simulink model "nonPred_TestModel_FCEV_ECMS_and_Battery_age"  (R2022b)
settings: Solver=ode4  StartTime=1  StopTime=DrvCycLen  FixedStep=Auto  RelTol=1e-3  EnableMultiTasking=on
values from neighbouring files (symbols this model uses):
  Bat_eff_chg_average = 0.969    [FCEV_original_data.mat]
  Bat_eff_dis_average = 0.9632    [FCEV_original_data.mat]
  Bat_end_of_life_percent = 20    [FCEV_original_data.mat]
  Bat_I_chg_max = -120    [FCEV_original_data.mat]
  Bat_I_dis_max = 200    [FCEV_original_data.mat]
  Bat_nom_Ic = 2.5    [FCEV_original_data.mat]
  Bat_nom_SOC = 0.35    [FCEV_original_data.mat]
  Bat_nom_temp_oC = 25    [FCEV_original_data.mat]
  Bat_num_pa = 9    [FCEV_original_data.mat]
  Bat_num_se = 97    [FCEV_original_data.mat]
  Bat_ori_C1_chg_F = [397.526659684 455.660832136 435.08783522 460.845064365 457.605812374 417.289828504 416.373906992 359.741413056 321.561704819 1109.14132554 1165.67733205 1135.97600211 ... (72 elements, 9x8)]    [FCEV_original_data.mat]
  Bat_ori_C1_dis_F = [187.121968588 287.083505726 346.448009002 395.529439835 387.517274826 389.973134196 432.856765051 486.92921923 512.158935268 425.990733989 614.68708868 771.472592368 ... (72 elements, 9x8)]    [FCEV_original_data.mat]
  Bat_ori_C2_chg_F = [8748.48589695 7773.35875681 9404.86567646 8934.73981058 8290.58671366 7592.78422269 7759.44623103 7396.59043829 6151.35152293 16187.7227039 11721.8480541 13157.8579836 ... (72 elements, 9x8)]    [FCEV_original_data.mat]
  Bat_ori_C2_dis_F = [2939.81325553 4590.73311898 5504.93546413 5887.5077374 6534.37836712 7765.46899768 10584.7751706 10372.0508438 9238.72693885 5207.86390693 7911.43744944 8879.62137571 ... (72 elements, 9x8)]    [FCEV_original_data.mat]
  Bat_ori_cap_max_Ah = 20.7    [Config_c221218.m]    (also in Config_c230117.m; Config_c230321.m; FCEV_original_data.mat)
  Bat_ori_dUdt4 = [-0.303773584906 -0.249056603774 -0.115094339623 -0.0396226415094 0.0396226415094 0.0641509433962 0.107547169811 0.111320754717 0.0415094339623 0.0547169811321 0.130188679245]    [FCEV_original_data.mat]
  Bat_ori_R0_chg_O = [0.0771669453735 0.0731809311402 0.0726556782939 0.0729965156794 0.0731758310684 0.0742031005051 0.0721266921026 0.0714211058078 0.0714186176143 0.0374124505155 0.0354566732504 0.0345430657188 ... (72 elements, 9x8)]    [FCEV_original_data.mat]
  Bat_ori_R0_dis_O = [0.0819458671157 0.0812429476608 0.0803749674507 0.0805513601722 0.0838629023857 0.0850797840015 0.0829875518672 0.0826388888889 0.0812514106148 0.0428124986417 0.0424658903711 0.0428572670451 ... (72 elements, 9x8)]    [FCEV_original_data.mat]
  Bat_ori_R1_chg_O = [0.114339870884 0.105392753268 0.104421193553 0.109821896183 0.114868279838 0.123333154908 0.129174812826 0.149917249373 0.174896487845 0.0420560161846 0.0390948352938 0.0370122837364 ... (72 elements, 9x8)]    [FCEV_original_data.mat]
  Bat_ori_R1_dis_O = [0.304806399643 0.213604089624 0.171463520004 0.151183840498 0.140630862434 0.128795299077 0.116857791733 0.112567113582 0.106368362501 0.0943235089866 0.0730697254134 0.0611414736086 ... (72 elements, 9x8)]    [FCEV_original_data.mat]
  Bat_ori_R2_chg_O = [0.134518959939 0.17565045702 0.161100627268 0.189032232545 0.205639040497 0.226170473035 0.223651875822 0.181765694192 0.212966950836 0.073628872144 0.0788540822416 0.0792414571734 ... (72 elements, 9x8)]    [FCEV_original_data.mat]
  Bat_ori_R2_dis_O = [0.354968099904 0.285293035102 0.286338708953 0.298763853987 0.248762838155 0.178586175471 0.129047399775 0.188406991173 0.174494800676 0.131839238891 0.123225430215 0.132069033134 ... (72 elements, 9x8)]    [FCEV_original_data.mat]
  Bat_ori_SOC2 = [0 0.001 0.002 0.003 0.004 0.005 0.006 0.007 0.008 0.009 0.01 0.011 ... (1001 elements, 1x1001)]    [FCEV_original_data.mat]
  Bat_ori_SOC4 = [-0.00598301069999 0.0920117618231 0.190864167279 0.289083557951 0.387343788287 0.485011843502 0.5850485992 0.678163031937 0.774810095565 0.876684636119 0.972739524626]    [FCEV_original_data.mat]
  Bat_ori_Uoc_chg_V = [2.4478 2.54923264342 2.6007 2.6383 2.66953057366 2.69636321708 2.7197 2.74042850391 2.75906114733 2.77619379074 2.792 2.80675907757 ... (1001 elements, 1x1001)]    [FCEV_original_data.mat]
  Bat_ori_Uoc_dis_V = [1.9998 2.03916768329 2.24724374236 2.39700902919 2.48767431602 2.5476 2.5882 2.6202 2.64771773167 2.6719 2.6933 2.71251566192 ... (1001 elements, 1x1001)]    [FCEV_original_data.mat]
  Bat_ori_Uoc_V = [2.2238 2.29420016335 2.42397187118 2.5176545146 2.57860244484 2.62198160854 2.65395 2.68031425195 2.7033894395 2.72404689537 2.74265 2.75963736975 ... (1001 elements, 1x1001)]    [FCEV_original_data.mat]
  Bat_single_capacity_nom_Ah = 2.3    [FCEV_original_data.mat]
  Bat_SOC_cs_max = 0.4    [FCEV_original_data.mat]
  Bat_SOC_cs_min = 0.2    [FCEV_original_data.mat]
  Bat_SOC_ini = 0.3    [Config_c22100601.m]    (also in Config_c22100701.m; FCEV_original_data.mat = 0.45)
  Bat_SOC_max = 0.9    [FCEV_original_data.mat]
  Bat_SOC_min = 0.3    [FCEV_original_data.mat]
  Bat_temp_amb_oC = 25    [FCEV_original_data.mat]
  Bat_temp_cool_oC = 25    [FCEV_original_data.mat]
  BattSocInit = 0.9    [Config_c221112.m]    (also in Config_c221127.m = 0.3; Config_c221218.m = 0.3; Config_c230117.m = 0.8; Config_c230321.m = 0.8)
  BattSocLowerLimit = 0.25    [Config_c221112.m]    (also in Config_c221127.m = 0.3; Config_c221218.m = 0.3; Config_c230117.m = 0.3; Config_c230321.m = 0.3)
  DCAC_eff = 0.95    [FCEV_original_data.mat]
  DCDC_ori_eff = [0.95 0.96 0.97 0.976 0.98 0.978 0.973 0.962]    [FCEV_original_data.mat]
  DCDC_ori_eff_avg = 0.9686    [FCEV_original_data.mat]
  DCDC_ori_power_kW = [0 10 20 30 40 50 60 70]    [FCEV_original_data.mat]
  FC_fuel_mass_ini_kg = 10    [FCEV_original_data.mat]
  FC_ori_eff = [0.1 0.33 0.492 0.533 0.559 0.596 0.591 0.562 0.508]    [FCEV_original_data.mat]
  FC_ori_fuel_rate_gps = [0 0.0505050505051 0.0846883468835 0.117260787992 0.149075730471 0.279642058166 0.423011844332 0.593119810202 0.820209973753]    [FCEV_original_data.mat]
  FC_ori_power_kW = [0 2 5 7.5 10 20 30 40 50]    [FCEV_original_data.mat]
  FC_power_max_kW = 50    [FCEV_original_data.mat]
  FC_power_min_kW = 0    [FCEV_original_data.mat]
  HydpriceRmb = 30    [Config_c221127.m]    (also in Config_c221218.m; Config_c230117.m; Config_c230321.m)
  m = Time_sample    [Config_c22100601.m]    (also in Config_c22100701.m)
  MC_eff_brk_average = 0.810578512397    [FCEV_original_data.mat]
  MC_eff_dri_average = 0.810578512397    [FCEV_original_data.mat]
  MC_inertia = 0.06    [FCEV_original_data.mat]
  MC_ori_eff = [0.7 0.78 0.85 0.86 0.81 0.82 0.79 0.78 0.78 0.78 0.78 0.7 ... (231 elements, 11x21)]    [FCEV_original_data.mat]
  MC_ori_power_brk_req_kW = [0 -28.3912930389 -56.7825860779 -85.1738791168 -113.565172156 -141.956465195 -170.347758234 -198.739051273 -227.130344311 -255.52163735 -283.912930389 0 ... (121 elements, 11x11)]    [FCEV_original_data.mat]
  MC_ori_power_dri_req_kW = [0 0 0 0 0 0 0 0 0 0 0 0 ... (121 elements, 11x11)]    [FCEV_original_data.mat]
  MC_ori_spd_rpm = [0 1000 2000 3000 4000 5000 6000 7000 8000 9000 10000]    [FCEV_original_data.mat]
  MC_ori_trq_brk_max_Nm = [-271.1368 -271.1368 -271.1368 -237.5159 -178.1369 -142.4824 -118.7579 -101.8119 -89.0685 -79.172 -71.1734]    [FCEV_original_data.mat]
  MC_ori_trq_brk_Nm = [-271.136848522 -244.02316367 -216.909478817 -189.795793965 -162.682109113 -135.568424261 -108.454739409 -81.3410545565 -54.2273697044 -27.1136848522 0]    [FCEV_original_data.mat]
  MC_ori_trq_dri_max_Nm = [271.1368 271.1368 271.1368 237.5159 178.1369 142.4824 118.7579 101.8119 89.0685 79.172 71.1734]    [FCEV_original_data.mat]
  MC_ori_trq_dri_Nm = [0 27.1136848522 54.2273697044 81.3410545565 108.454739409 135.568424261 162.682109113 189.795793965 216.909478817 244.02316367 271.136848522]    [FCEV_original_data.mat]
  MC_ori_trq_Nm = [-271.136848522 -244.02316367 -216.909478817 -189.795793965 -162.682109113 -135.568424261 -108.454739409 -81.3410545565 -54.2273697044 -27.1136848522 0 27.1136848522 ... (21 elements, 1x21)]    [FCEV_original_data.mat]
  MC_power_max_kW = 75    [FCEV_original_data.mat]
  MC_spd_max_rpm = 10000    [FCEV_original_data.mat]
  MC_spd_min_rpm = 0    [FCEV_original_data.mat]
  MC_spd_scale = 1    [FCEV_original_data.mat]
  MC_trq_scale = 1    [FCEV_original_data.mat]
  MC_U_min_V = 120    [FCEV_original_data.mat]
  Road_u = 0.75    [FCEV_original_data.mat]
  tDegTable = [zeros(1,3),linspace(0,0.13,47)]    [Config_c221127.m]    (also in Config_c221218.m; Config_c230117.m; Config_c230321.m)
  usd2rmb = 7.116    [Config_c22100601.m]    (also in Config_c22100701.m; Config_c221106.m = 6; Config_c221112.m = 6; Config_c221127.m = 6)
  Veh_air_density_kgpm2 = 1.2    [FCEV_original_data.mat]
  Veh_brk_front = [1 0.6 0.608 0.61 0.618 0.624 0.636 0.645 0.655]    [FCEV_original_data.mat]
  Veh_brk_z = [0.1 0.2 0.3 0.4 0.5 0.6 0.7 0.8 0.9]    [FCEV_original_data.mat]
  Veh_brk_z_max = 0.7    [FCEV_original_data.mat]
  Veh_brk_z_min = 0.1    [FCEV_original_data.mat]
  Veh_coeff_drag = 0.312    [FCEV_original_data.mat]
  Veh_coeff_roll = 0.00863    [FCEV_original_data.mat]
  Veh_final_drive_inertia = 0.1105    [FCEV_original_data.mat]
  Veh_final_drive_ratio = 3.47    [FCEV_original_data.mat]
  Veh_frontal_area_m2 = 2.06    [FCEV_original_data.mat]
  Veh_gravity_acc_ms2 = 9.81    [FCEV_original_data.mat]
  Veh_mass_cargo_kg = 113    [FCEV_original_data.mat]
  Veh_mass_curb_kg = 1157    [FCEV_original_data.mat]
  Veh_mech_eff = 0.9    [FCEV_original_data.mat]
  Veh_rotary_mass_conversion_factor = 1.05    [FCEV_original_data.mat]
  Veh_size_cg_height_m = 0.53    [FCEV_original_data.mat]
  Veh_wheel_inertia = 3.1039    [FCEV_original_data.mat]
  Veh_wheel_radius_m = 0.313    [FCEV_original_data.mat]
  Veh_wt_frac_front = 0.5    [FCEV_original_data.mat]
undefined symbols (not defined in the file or in its folder): Bat_ori_temp
libraries: autolibshared x1
(part 1 of 3)
settings Model: Creator=阿瑞的PC  LastModifiedBy=xuupp
settings SolverCC: AlgebraicLoopSolver=TrustRegion
settings DataIOCC: LimitDataPoints=on  SaveFormat=Array  ReturnWorkspaceOutputs=off
settings OptimizationCC: LifeSpan=inf
settings DebuggingCC: MaxConsecutiveZCsMsg=none  SolverPrmCheckMsg=warning  UnconnectedInputMsg=warning  UnconnectedOutputMsg=warning  UnconnectedLineMsg=warning  SFUnexpectedBacktrackingDiag=warning  SFNoUnconditionalDefaultTransitionDiag=warning  SFExecutionAtInitializationDiag=none  SFMachineParentedDataDiag=warning  ArithmeticOperatorsInVariantConditions=warning
settings HardwareCC: ProdBitPerPointer=32  ProdBitPerSizeT=32  ProdBitPerPtrDiffT=32  ProdLargestAtomicFloat=None  ProdIntDivRoundTo=Undefined  ProdEndianess=Unspecified  ProdWordSize=32  ProdHWDeviceType=32-bit Generic
settings ModelReferenceCC: EnableRefExpFcnMdlSchedulingChecks=on  PropagateSignalLabelsOutOfModel=off
settings SFSimCC: SimUseLocalCustomCode=off  CustomCodeUndefinedFunction=UseInterfaceOnly
settings RTWCC: RTWUseLocalCustomCode=off  DLArmComputeVersion=19.05
settings CodeAppCC: StateflowObjectComments=on
settings GRTTargetCC: TargetLangStandard=C89/C90 (ANSI)
settings ConfigComp: CovMetricSettings=dw  CovSaveCumulativeToWorkspaceVar=on  CovSaveSingleToWorkspaceVar=on  CovExternalEMLEnable=off  CovSFcnEnable=off
settings SimscapeCC: SimscapeNormalizeSystem=off
settings ConfigurationSet: Description=SimMechanics 2G

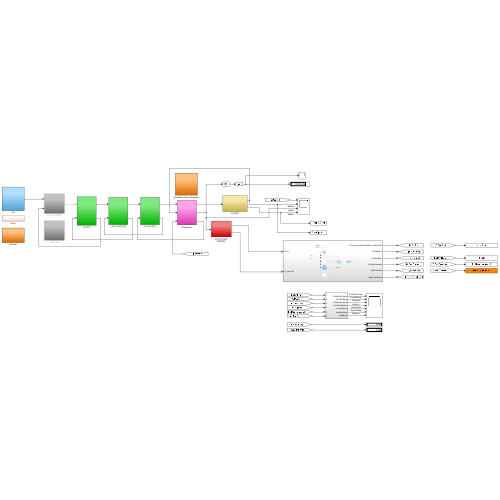
[thumbnail: Simulink's stored preview of the top-level diagram]
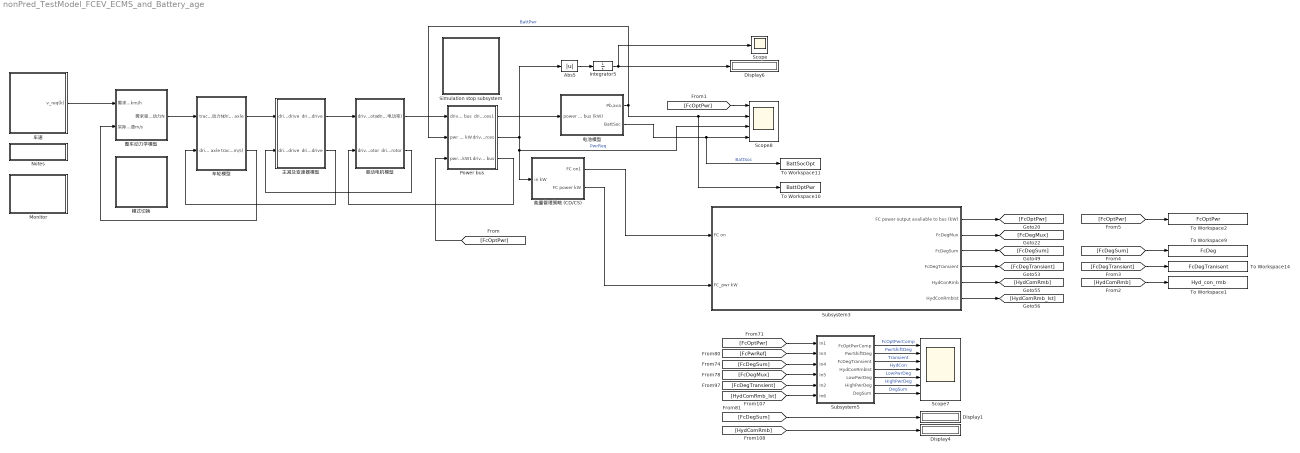
== system nonPred_TestModel_FCEV_ECMS_and_Battery_age ==
  Abs5 : Abs  SaturateOnIntegerOverflow=off
  Display1 : Display
  Display4 : Display
  Display6 : Display
  Integrator5 : Integrator
  Monitor : Subsystem
  Notes : Subsystem
  Power bus : Subsystem
  Scope : Scope
  Scope7 : Scope  NumInputPorts=7
  Scope8 : Scope  NumInputPorts=4
  Simulation stop subsystem : Subsystem
  Subsystem3 : Subsystem
  Subsystem5 : Subsystem
  To Workspace1 : ToWorkspace  VariableName=Hyd_con_rmb  SampleTime=-1
  To Workspace10 : ToWorkspace  VariableName=BattOptPwr  SampleTime=-1
  To Workspace11 : ToWorkspace  VariableName=BattSocOpt  SampleTime=-1
  To Workspace14 : ToWorkspace  VariableName=FcDegTranisent  SampleTime=-1
  To Workspace2 : ToWorkspace  VariableName=FcOptPwr  SampleTime=-1
  To Workspace9 : ToWorkspace  VariableName=FcDeg  SampleTime=-1
  主减及变速器模型 : Subsystem
  整车动力学模型 : Subsystem
  模式切换 : Subsystem
  电池模型 : Subsystem
  能量管理策略 (CD/CS) : Subsystem
  车轮模型 : Subsystem
  车速 : Subsystem
  驱动电机模型 : Subsystem
  wires:
  主减及变速器模型/1(drive torque (Nm) speed (rad/s) brike torque (Nm) req'd at input side of final drive) -> 驱动电机模型/1(drive torque (Nm) speed (rad/s) brake torque (Nm) req'd at motor)
  驱动电机模型/2(drive torque (Nm) brake torque (Nm) speed avail (rad/s) avail. at rotor) -> 主减及变速器模型/2(drive torque (Nm) brake torque (Nm) speed avail (rad/s) at input side of final drive)
  主减及变速器模型/2(drive torque (Nm) brake torque (Nm) speed avail (rad/s) at output side of final drive) -> 车轮模型/2("drive torque (Nm) brake torque (Nm) speed (rad/s) available from drivetrain into axle ")
  车轮模型/2(tractive force (N) brake force (N) linear speed achievable (m/s)) -> 整车动力学模型/2(实际车辆驱动力N 制动力N 和车速m/s)
  整车动力学模型/1(需求驱动力N 目标车速m/s 需求制动力N) -> 车轮模型/1("tractive force, brake force and speed req'd of tire/road interface 需求驱动力N 目标车速m/s 需求制动力N")
  电池模型/1(Pb,ava) -> To Workspace10/1, Scope8/2, Power bus/2(pwr availible from battery kW)  "BattPwr"
  车轮模型/1(drive torque (Nm) speed (rad/s) brake torque (Nm) req'd from drivetrain into axle) -> 主减及变速器模型/1(drive torque (Nm) speed (rad/s) brake torque (Nm) req'd at output side of final drive)
  车速/1(v_req(k)) -> 整车动力学模型/1(需求车速 km/h)
  能量管理策略 (CD/CS)/2(FC power kW) -> Subsystem3/2("FC_pwr kW ")
  能量管理策略 (CD/CS)/1(FC on1) -> Subsystem3/1(FC on)
  Power bus/1(drive power (kW)/brake power (kW) req from power sources1) -> 电池模型/1(power req'd into bus (kW))
  Power bus/3(drive power (kW) brake power (kW) availableat power bus) -> 驱动电机模型/2(drive power (kW) brake power (kW) input available motor)
  Power bus/2(drive power (kW)/brake power (kW) req from power sources) -> Scope8/3, 能量管理策略 (CD/CS)/1(in kW), Abs5/1  "PwrReq"
  驱动电机模型/1(drive power (kW) brake power (kW) req'd motor input power (电功率)) -> Power bus/1(drive power (kW) brake power (kW) req at power bus)
  Abs5/1 -> Integrator5/1
  Integrator5/1 -> Display6/1, Scope/1
  电池模型/2(BattSoc) -> To Workspace11/1, Scope8/4  "BattSoc"
  Subsystem3/6(HydConRmbIst) -> [HydComRmb_Ist]
  Subsystem3/5(HydConRmb) -> [HydComRmb]
  Subsystem3/4(FcDegTransient) -> [FcDegTransient]
  Subsystem3/2(FcDegMux) -> [FcDegMux]
  Subsystem3/1(FC power output avaliable to bus (kW)) -> [FcOptPwr]
  Subsystem3/3(FcDegSum) -> [FcDegSum]
  [FcOptPwr] -> Power bus/3(pwr availible from FC kW1)
  [FcOptPwr] -> Scope8/1
  [FcOptPwr] -> Subsystem5/1(In1)
  [HydComRmb_Ist] -> Subsystem5/6(In6)
  [FcDegTransient] -> Subsystem5/5(In2)
  Subsystem5/5(LowPwrDeg) -> Scope7/5  "LowPwrDeg"
  Subsystem5/7(DegSum) -> Scope7/7  "DegSum"
  Subsystem5/2(PwrShiftDeg) -> Scope7/2  "PwrShiftDeg"
  Subsystem5/4(HydConRmbIst) -> Scope7/4  "HydCon"
  Subsystem5/6(HighPwrDeg) -> Scope7/6  "HighPwrDeg"
  [FcDegMux] -> Subsystem5/4(In5)
  [FcPwrRef] -> Subsystem5/2(In3)
  Subsystem5/3(FcDegTransient) -> Scope7/3  "Transient"
  [FcDegSum] -> Subsystem5/3(In4)
  Subsystem5/1(FcOptPwrComp) -> Scope7/1  "FcOptPwrComp"
  [HydComRmb] -> Display4/1
  [FcDegSum] -> Display1/1
  [HydComRmb] -> To Workspace1/1
  [FcDegTransient] -> To Workspace14/1
  [FcDegSum] -> To Workspace9/1
  [FcOptPwr] -> To Workspace2/1

== system nonPred_TestModel_FCEV_ECMS_and_Battery_age/Monitor ==
  note: 燃料电池模块
  note: 电池模块
  note: Power bus
  note: 电机模块
  note: 车速模块
  Display{,1..7} (8 alike) : Display
  Scope : Scope
  wires:
  [Trip_distance_travelled_km] -> Display/1
  [MC_power_dri_req_kW] -> Display1/1
  [MC_power_brk_req_kW] -> Display2/1
  [PS_power_req_kW] -> Display3/1
  [Bat_charge_sustaining_on] -> Display4/1
  [Bat_SOC] -> Scope/1, Display5/1
  [FC_fuel_rate_gps] -> Display6/1
  [FC_fuel_consume_kg] -> Display7/1

== system nonPred_TestModel_FCEV_ECMS_and_Battery_age/Notes ==
  note: Notes:
      | #1:涉及单位换算的模块统一使用紫色底色；

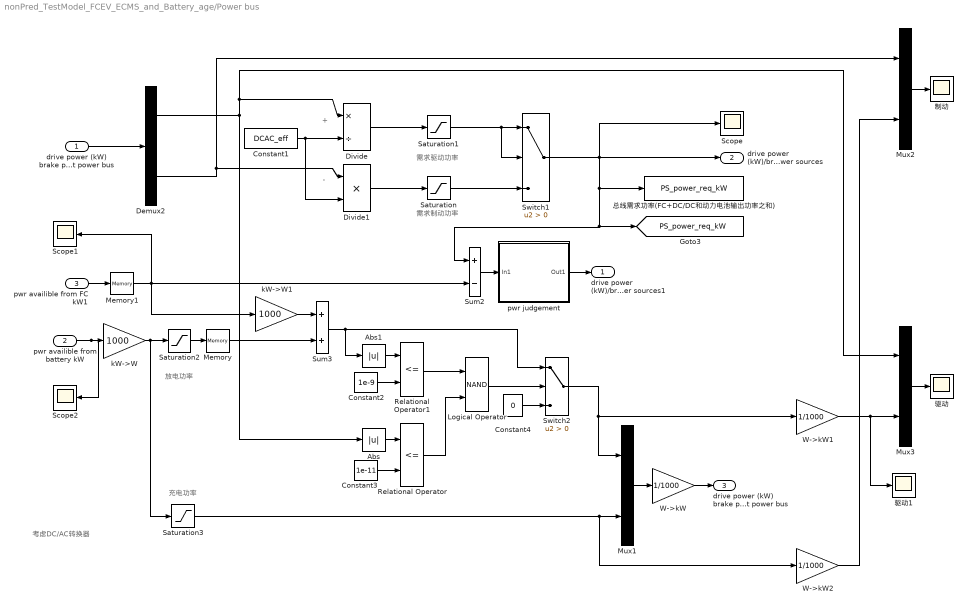
== system nonPred_TestModel_FCEV_ECMS_and_Battery_age/Power bus ==
  note: 充电功率
  note: 放电功率
  note: 考虑DC/AC转换器
  note: -
  note: +
  note: 需求制动功率
  note: 需求驱动功率
  drive power (kW) brake power (kW) req at power bus : Inport
  pwr availible from battery kW : Inport  Port=2
  pwr availible from FC kW1 : Inport  Port=3
  Abs : Abs  SaturateOnIntegerOverflow=off
  Abs1 : Abs  SaturateOnIntegerOverflow=off
  Constant1 : Constant  Value=DCAC_eff
  Constant2 : Constant  Value=1e-9
  Constant3 : Constant  Value=1e-11
  Constant4 : Constant  Value=0
  Demux2 : Demux  Outputs=2
  Divide : Product  Inputs=*/
  Divide1 : Product  Inputs=**
  Logical Operator : Logic  Operator=NAND  AllPortsSameDT=off  OutDataTypeStr=boolean
  Memory : Memory  InheritSampleTime=on
  Memory1 : Memory  InheritSampleTime=on
  Mux1 : Mux  Inputs=2
  Mux2 : Mux  Inputs=2
  Mux3 : Mux  Inputs=2
  Relational Operator : RelationalOperator  Operator=<=  OutDataTypeStr=boolean  InputSameDT=off
  Relational Operator1 : RelationalOperator  Operator=<=  OutDataTypeStr=boolean  InputSameDT=off
  Saturation : Saturate  UpperLimit=0  LowerLimit=-inf
  Saturation1 : Saturate  UpperLimit=inf  LowerLimit=0
  Saturation2 : Saturate  UpperLimit=inf  LowerLimit=0
  Saturation3 : Saturate  UpperLimit=0  LowerLimit=-inf
  Scope : Scope
  Scope1 : Scope
  Scope2 : Scope
  Sum2 : Sum  Inputs=+-
  Sum3 : Sum
  Switch1 : Switch  Criteria=u2 > Threshold  SaturateOnIntegerOverflow=off  InputSameDT=off
  Switch2 : Switch  Criteria=u2 > Threshold  SaturateOnIntegerOverflow=off  InputSameDT=off
  W->kW : Gain  Gain=1/1000
  W->kW1 : Gain  Gain=1/1000
  W->kW2 : Gain  Gain=1/1000
  kW->W : Gain  Gain=1000
  kW->W1 : Gain  Gain=1000
  pwr judgement : Subsystem
  制动 : Scope
  总线需求功率(FC+DC/DC和动力电池输出功率之和) : ToWorkspace  VariableName=PS_power_req_kW  SampleTime=-1
  驱动 : Scope
  驱动1 : Scope
  drive power (kW)/brake power (kW) req from power sources1 : Outport
  drive power (kW)/brake power (kW) req from power sources : Outport  Port=2
  drive power (kW) brake power (kW) availableat power bus : Outport  Port=3
  tag scope: PS_power_req_kW=global
  wires:
  Abs1/1 -> Relational Operator1/1
  Constant2/1 -> Relational Operator1/2
  Constant1/1 -> Divide1/2, Divide/2
  Divide/1 -> Saturation1/1
  Divide1/1 -> Saturation/1
  drive power (kW) brake power (kW) req at power bus/1 -> Demux2/1
  Demux2/2 -> Mux2/1, Divide1/1
  Saturation1/1 -> Switch1/2, Switch1/1
  Switch1/1 -> drive power (kW)/brake power (kW) req from power sources/1, 总线需求功率(FC+DC/DC和动力电池输出功率之和)/1, Sum2/1, [PS_power_req_kW], Scope/1
  W->kW/1 -> drive power (kW) brake power (kW) availableat power bus/1
  Saturation/1 -> Switch1/3
  Mux2/1 -> 制动/1
  Mux3/1 -> 驱动/1
  W->kW1/1 -> 驱动1/1, Mux3/2
  W->kW2/1 -> Mux2/2
  Sum2/1 -> pwr judgement/1(In1)
  pwr judgement/1(Out1) -> drive power (kW)/brake power (kW) req from power sources1/1
  Saturation2/1 -> Memory/1
  Memory/1 -> Sum3/2
  Memory1/1 -> kW->W1/1, Scope1/1, Sum2/2
  Sum3/1 -> Switch2/1, Abs1/1
  Relational Operator1/1 -> Logical Operator/1
  Abs/1 -> Relational Operator/1
  Constant3/1 -> Relational Operator/2
  Demux2/1 -> Mux3/1, Divide/1, Abs/1
  Relational Operator/1 -> Logical Operator/2
  Constant4/1 -> Switch2/3
  Logical Operator/1 -> Switch2/2
  Saturation3/1 -> W->kW2/1, Mux1/2
  Switch2/1 -> W->kW1/1, Mux1/1
  pwr availible from battery kW/1 -> Scope2/1, kW->W/1
  kW->W/1 -> Saturation3/1, Saturation2/1
  kW->W1/1 -> Sum3/1
  Mux1/1 -> W->kW/1
  pwr availible from FC kW1/1 -> Memory1/1

== system nonPred_TestModel_FCEV_ECMS_and_Battery_age/Simulation stop subsystem ==
  note: 能量不足停止仿真
  note: 到达终点停止仿真
  . : Constant  Value=FC_fuel_mass_ini_kg
  ... : Integrator
  .1 : Constant  Value=139.3
  .2 : Constant  Value=0
  Constant1 : Constant  Value=Bat_SOC_min
  Display3 : Display
  Gain : Gain  Gain=1/1000
  Logical Operator : Logic  AllPortsSameDT=off  OutDataTypeStr=boolean
  Relational Operator1 : RelationalOperator  Operator=<=  OutDataTypeStr=boolean  InputSameDT=off
  Relational Operator2 : RelationalOperator
  Relational Operator3 : RelationalOperator
  Saturation : Saturate  UpperLimit=1  LowerLimit=-1
  Stop Simulation : Stop
  Stop Simulation1 : Stop
  Switch : Switch  Criteria=u2 > Threshold
  wires:
  [Bat_SOC] -> Relational Operator1/1
  Constant1/1 -> Relational Operator1/2
  Relational Operator1/1 -> Logical Operator/2
  Logical Operator/1 -> Stop Simulation/1
  Relational Operator2/1 -> Logical Operator/1
  ./1 -> Relational Operator2/2
  [Trip_distance_travelled_km] -> Relational Operator3/1, Display3/1
  .1/1 -> Relational Operator3/2
  Relational Operator3/1 -> Stop Simulation1/1
  [FC_on] -> Switch/2
  .2/1 -> Switch/3
  Switch/1 -> .../1
  [FC_fuel_rate_gps] -> Saturation/1
  Saturation/1 -> Switch/1
  .../1 -> Gain/1
  Gain/1 -> Relational Operator2/1

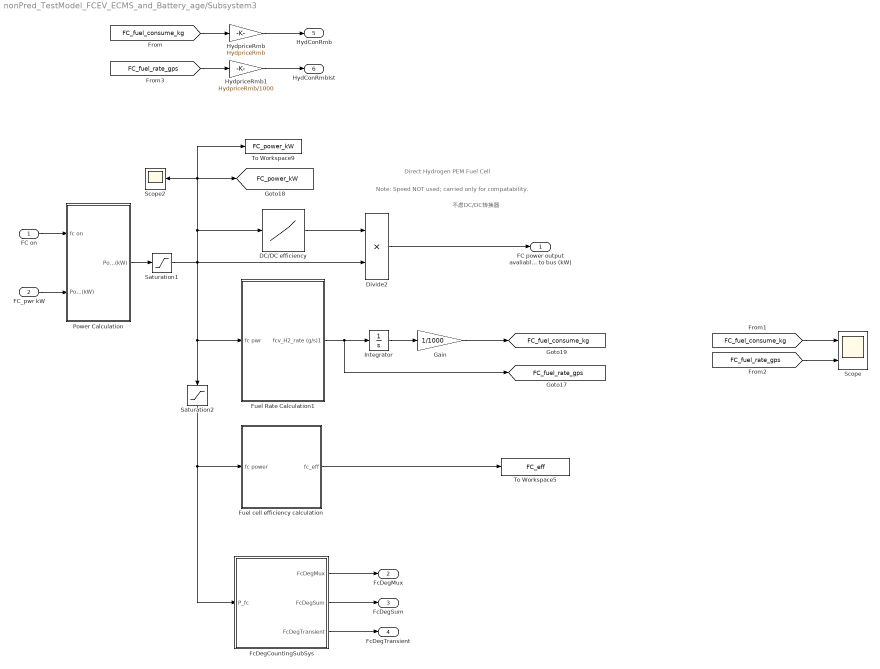
== system nonPred_TestModel_FCEV_ECMS_and_Battery_age/Subsystem3 ==
  note: Direct Hydrogen PEM Fuel Cell
  note: Note: Speed NOT used; carried only for compatability.
  note: 不虑DC/DC转换器
  FC on : Inport
  "FC_pwr kW " : Inport  Port=2
  DC/DC efficiency : Lookup_n-D  NumberOfTableDimensions=1  BreakpointsForDimension1=DCDC_ori_power_kW  Table=DCDC_ori_eff  RndMeth=Simplest
  Divide2 : Product  Inputs=**
  FcDegCountingSubSys : Subsystem
  Fuel Rate Calculation1 : Subsystem
  Fuel cell efficiency calculation : Subsystem
  Gain : Gain  Gain=1/1000
  HydpriceRmb : Gain  Gain=HydpriceRmb
  HydpriceRmb1 : Gain  Gain=HydpriceRmb/1000
  Integrator : Integrator
  Power Calculation : Subsystem
  Saturation1 : Saturate  UpperLimit=FC_power_max_kW  LowerLimit=FC_power_min_kW
  Saturation2 : Saturate  UpperLimit=FC_power_max_kW  LowerLimit=FC_power_min_kW
  Scope : Scope  NumInputPorts=2
  Scope2 : Scope
  To Workspace5 : ToWorkspace  VariableName=FC_eff  SampleTime=-1
  To Workspace9 : ToWorkspace  VariableName=FC_power_kW  SampleTime=-1
  FC power output avaliable to bus (kW) : Outport
  FcDegMux : Outport  Port=2
  FcDegSum : Outport  Port=3
  FcDegTransient : Outport  Port=4
  HydConRmb : Outport  Port=5
  HydConRmbIst : Outport  Port=6
  tag scope: FC_fuel_consume_kg=global, FC_fuel_rate_gps=global, FC_power_kW=global
  wires:
  Saturation2/1 -> FcDegCountingSubSys/1(P_fc), Fuel cell efficiency calculation/1(fc power)
  Divide2/1 -> FC power output avaliable to bus (kW)/1
  Fuel Rate Calculation1/1(fcv_H2_rate (g/s)1) -> Integrator/1, [FC_fuel_rate_gps]
  Fuel cell efficiency calculation/1("fc_eff ") -> To Workspace5/1
  Saturation1/1 -> DC/DC efficiency/1, Scope2/1, [FC_power_kW], To Workspace9/1, Divide2/2, Saturation2/1, Fuel Rate Calculation1/1(fc pwr)
  FcDegCountingSubSys/2(FcDegSum) -> FcDegSum/1
  FcDegCountingSubSys/1(FcDegMux) -> FcDegMux/1
  DC/DC efficiency/1 -> Divide2/1
  Gain/1 -> [FC_fuel_consume_kg]
  FC on/1 -> Power Calculation/1(fc on)
  Power Calculation/1(Power output (kW)) -> Saturation1/1
  "FC_pwr kW "/1 -> Power Calculation/2(Power command (kW))
  Integrator/1 -> Gain/1
  FcDegCountingSubSys/3(FcDegTransient) -> FcDegTransient/1
  [FC_fuel_consume_kg] -> HydpriceRmb/1
  [FC_fuel_rate_gps] -> Scope/2
  [FC_fuel_consume_kg] -> Scope/1
  HydpriceRmb/1 -> HydConRmb/1
  [FC_fuel_rate_gps] -> HydpriceRmb1/1
  HydpriceRmb1/1 -> HydConRmbIst/1

== system nonPred_TestModel_FCEV_ECMS_and_Battery_age/Subsystem5 ==
  In1 : Inport
  In3 : Inport  Port=2
  In4 : Inport  Port=3
  In5 : Inport  Port=4
  In2 : Inport  Port=5
  In6 : Inport  Port=6
  Demux2 : Demux  Outputs=3
  Mux4 : Mux  Inputs=2
  FcOptPwrComp : Outport
  PwrShiftDeg : Outport  Port=2
  FcDegTransient : Outport  Port=3
  HydConRmbIst : Outport  Port=4
  LowPwrDeg : Outport  Port=5
  HighPwrDeg : Outport  Port=6
  DegSum : Outport  Port=7
  wires:
  Mux4/1 -> FcOptPwrComp/1
  Demux2/2 -> LowPwrDeg/1  "LowPwrDeg"
  Demux2/3 -> PwrShiftDeg/1  "PwrShiftDeg"
  Demux2/1 -> HighPwrDeg/1  "HighPwrDeg"
  In4/1 -> DegSum/1  "FcDegSum"
  In3/1 -> Mux4/2  "Ref"
  In1/1 -> Mux4/1  "Opt"
  In5/1 -> Demux2/1
  In2/1 -> FcDegTransient/1
  In6/1 -> HydConRmbIst/1

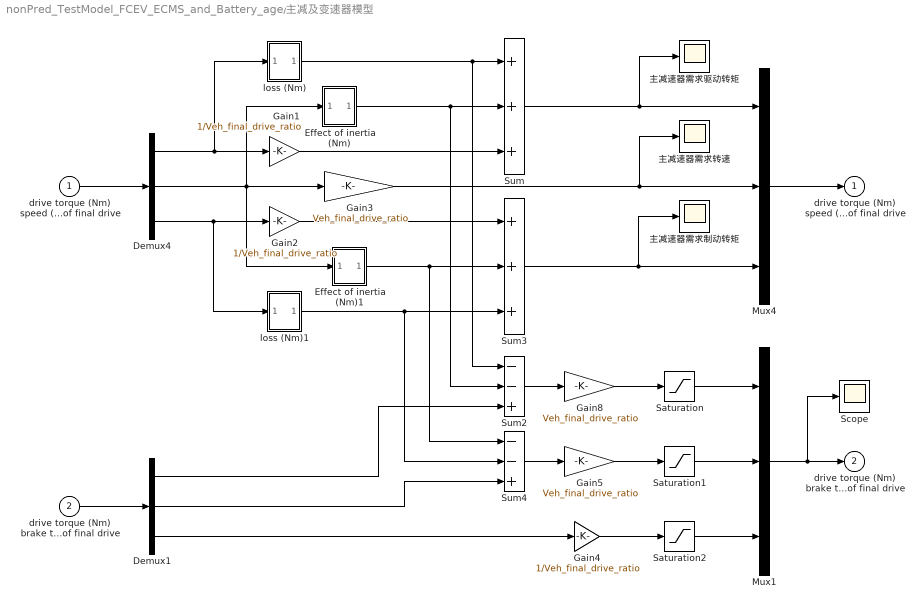
== system nonPred_TestModel_FCEV_ECMS_and_Battery_age/主减及变速器模型 ==
  drive torque (Nm) speed (rad/s) brake torque (Nm) req'd at output side of final drive : Inport
  drive torque (Nm) brake torque (Nm) speed avail (rad/s) at input side of final drive : Inport  Port=2
  " Effect of inertia (Nm)1" : Subsystem
  Demux1 : Demux  Outputs=3
  Demux4 : Demux  Outputs=3
  Effect of inertia (Nm) : Subsystem
  Gain1 : Gain  Gain=1/Veh_final_drive_ratio
  Gain2 : Gain  Gain=1/Veh_final_drive_ratio
  Gain3 : Gain  Gain=Veh_final_drive_ratio  SaturateOnIntegerOverflow=on  OutDataTypeStr=Inherit: Same as input  ParamDataTypeStr=Inherit: Same as input
  Gain4 : Gain  Gain=1/Veh_final_drive_ratio  SaturateOnIntegerOverflow=on  OutDataTypeStr=Inherit: Same as input  ParamDataTypeStr=Inherit: Same as input
  Gain5 : Gain  Gain=Veh_final_drive_ratio  SaturateOnIntegerOverflow=on  OutDataTypeStr=Inherit: Same as input  ParamDataTypeStr=Inherit: Same as input
  Gain8 : Gain  Gain=Veh_final_drive_ratio  SaturateOnIntegerOverflow=on  OutDataTypeStr=Inherit: Same as input  ParamDataTypeStr=Inherit: Same as input
  Mux1 : Mux  Inputs=3
  Mux4 : Mux  Inputs=3
  Saturation : Saturate  UpperLimit=inf  LowerLimit=0
  Saturation1 : Saturate  UpperLimit=0  LowerLimit=-inf
  Saturation2 : Saturate  UpperLimit=inf  LowerLimit=0
  Scope : Scope
  Sum : Sum  Inputs=+++  InputSameDT=on  SaturateOnIntegerOverflow=on  OutDataTypeStr=Inherit: Same as first input
  Sum2 : Sum  Inputs=--+  InputSameDT=on  SaturateOnIntegerOverflow=on  OutDataTypeStr=Inherit: Same as first input
  Sum3 : Sum  Inputs=+++  InputSameDT=on  SaturateOnIntegerOverflow=on  OutDataTypeStr=Inherit: Same as first input
  Sum4 : Sum  Inputs=--+  InputSameDT=on  SaturateOnIntegerOverflow=on  OutDataTypeStr=Inherit: Same as first input
  loss (Nm) : Subsystem
  loss (Nm)1 : Subsystem
  主减速器需求制动转矩 : Scope
  主减速器需求转速 : Scope
  主减速器需求驱动转矩 : Scope
  drive torque (Nm) speed (rad/s) brike torque (Nm) req'd at input side of final drive : Outport  InitialOutput=0
  drive torque (Nm) brake torque (Nm) speed avail (rad/s) at output side of final drive : Outport  Port=2  InitialOutput=0
  wires:
  Demux4/2 -> Effect of inertia (Nm)/1(fd input speed (rad/s)), " Effect of inertia (Nm)1"/1(In1), Gain3/1
  Demux4/1 -> loss (Nm)/1("drive torque (Nm) "), Gain1/1
  Mux4/1 -> drive torque (Nm) speed (rad/s) brike torque (Nm) req'd at input side of final drive/1
  drive torque (Nm) speed (rad/s) brake torque (Nm) req'd at output side of final drive/1 -> Demux4/1
  Mux1/1 -> Scope/1, drive torque (Nm) brake torque (Nm) speed avail (rad/s) at output side of final drive/1
  drive torque (Nm) brake torque (Nm) speed avail (rad/s) at input side of final drive/1 -> Demux1/1
  Effect of inertia (Nm)/1(drag torque (Nm)) -> Sum2/2, Sum/2
  loss (Nm)/1(drag torque (Nm)) -> Sum2/1, Sum/1
  Gain1/1 -> Sum/3
  Sum/1 -> 主减速器需求驱动转矩/1, Mux4/1
  Gain3/1 -> 主减速器需求转速/1, Mux4/2
  " Effect of inertia (Nm)1"/1(Out1) -> Sum4/1, Sum3/2
  loss (Nm)1/1(drag torque (Nm)) -> Sum4/2, Sum3/3
  Demux4/3 -> Gain2/1, loss (Nm)1/1("drive torque (Nm) ")
  Gain2/1 -> Sum3/1
  Demux1/1 -> Sum2/3
  Demux1/2 -> Sum4/3
  Sum2/1 -> Gain8/1
  Gain8/1 -> Saturation/1
  Saturation/1 -> Mux1/1
  Sum4/1 -> Gain5/1
  Saturation1/1 -> Mux1/2
  Gain5/1 -> Saturation1/1
  Gain4/1 -> Saturation2/1
  Demux1/3 -> Gain4/1
  Saturation2/1 -> Mux1/3
  Sum3/1 -> 主减速器需求制动转矩/1, Mux4/3

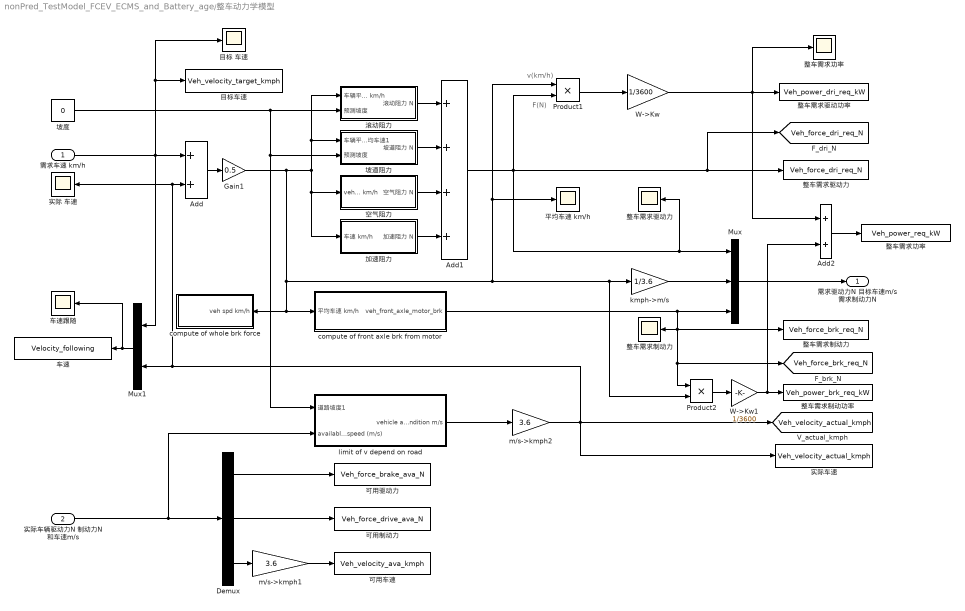
== system nonPred_TestModel_FCEV_ECMS_and_Battery_age/整车动力学模型 ==
  note: v(km/h)
  note: F(N)
  需求车速 km/h : Inport
  实际车辆驱动力N 制动力N 和车速m/s : Inport  Port=2
  "  整车需求制动力" : ToWorkspace  VariableName=Veh_force_brk_req_N  SaveFormat=Timeseries  SampleTime=-1
  "  整车需求制动功率" : ToWorkspace  VariableName=Veh_power_brk_req_kW  SampleTime=-1
  "  整车需求功率" : ToWorkspace  VariableName=Veh_power_req_kW  SampleTime=-1
  "  整车需求驱动力" : ToWorkspace  VariableName=Veh_force_dri_req_N  SaveFormat=Timeseries  SampleTime=-1
  "  整车需求驱动功率" : ToWorkspace  VariableName=Veh_power_dri_req_kW  SampleTime=-1
  "  目标车速" : ToWorkspace  VariableName=Veh_velocity_target_kmph  SaveFormat=Timeseries  SampleTime=-1
  "  车速" : ToWorkspace  VariableName=Velocity_following  SaveFormat=Timeseries  SampleTime=-1
  Add : Sum
  Add1 : Sum  Inputs=++++
  Add2 : Sum
  Demux : Demux  Outputs=3
  Gain1 : Gain  Gain=0.5
  Mux : Mux  Inputs=3
  Mux1 : Mux  Inputs=2
  Product1 : Product  RndMeth=Zero
  Product2 : Product  RndMeth=Zero
  W->Kw : Gain  Gain=1/3600
  W->Kw1 : Gain  Gain=1/3600
  compute of front axle brk from motor : Subsystem
  compute of whole brk force : Subsystem
  kmph->m/s : Gain  Gain=1/3.6
  limit of v depend on road : Subsystem
  m/s->kmph1 : Gain  Gain=3.6
  m/s->kmph2 : Gain  Gain=3.6
  加速阻力 : Subsystem
  可用制动力 : ToWorkspace  VariableName=Veh_force_drive_ava_N  SaveFormat=Timeseries  SampleTime=-1
  可用车速 : ToWorkspace  VariableName=Veh_velocity_ava_kmph  SaveFormat=Timeseries  SampleTime=-1
  可用驱动力 : ToWorkspace  VariableName=Veh_force_brake_ava_N  SaveFormat=Timeseries  SampleTime=-1
  坡度 : Constant  Value=0
  坡道阻力 : Subsystem
  实际 车速 : Scope
  实际车速 : ToWorkspace  VariableName=Veh_velocity_actual_kmph  SaveFormat=Timeseries  SampleTime=-1
  平均车速 km/h : Scope
  整车需求制动力 : Scope
  整车需求功率 : Scope
  整车需求驱动力 : Scope
  滚动阻力 : Subsystem
  目标 车速 : Scope
  空气阻力 : Subsystem
  车速跟随 : Scope
  需求驱动力N 目标车速m/s 需求制动力N : Outport
  tag scope: Veh_force_brk_req_N=global, Veh_force_dri_req_N=global, Veh_velocity_actual_kmph=global
  wires:
  需求车速 km/h/1 -> Mux1/1, Add/1, 目标 车速/1, "  目标车速"/1
  Add/1 -> Gain1/1
  实际车辆驱动力N 制动力N 和车速m/s/1 -> limit of v depend on road/2(available drive force (N) brake force (N) and linear speed (m/s)), Demux/1
  滚动阻力/1(滚动阻力 N) -> Add1/1
  坡道阻力/1(坡道阻力 N) -> Add1/2
  空气阻力/1(空气阻力 N) -> Add1/3
  加速阻力/1(加速阻力 N) -> Add1/4
  Add1/1 -> 整车需求驱动力/1, Mux/1, [Veh_force_dri_req_N], "  整车需求驱动力"/1, Product1/2
  Mux/1 -> 需求驱动力N 目标车速m/s 需求制动力N/1
  Product1/1 -> W->Kw/1
  Demux/1 -> 可用驱动力/1
  坡度/1 -> limit of v depend on road/1(道路坡度1), 坡道阻力/2(预测坡度), 滚动阻力/2(预测坡度)
  W->Kw/1 -> 整车需求功率/1, Add2/1, "  整车需求驱动功率"/1
  kmph->m/s/1 -> Mux/2
  limit of v depend on road/1(vehicle achievable consider of the road condition m/s) -> m/s->kmph2/1
  m/s->kmph2/1 -> 实际车速/1, Mux1/2, 实际 车速/1, Add/2, [Veh_velocity_actual_kmph]
  Gain1/1 -> compute of front axle brk from motor/1(平均车速 km/h), compute of whole brk force/1(veh spd km/h), Product2/2, kmph->m/s/1, 平均车速 km/h/1, Product1/1, 加速阻力/1(车速 km/h), 空气阻力/1(veh_spd km/h), 滚动阻力/1(车辆平均车速 km/h), 坡道阻力/1(车辆平均车速1)
  m/s->kmph1/1 -> 可用车速/1
  compute of front axle brk from motor/1(veh_front_axle_motor_brk) -> Mux/3, 整车需求制动力/1, "  整车需求制动力"/1, [Veh_force_brk_req_N], Product2/1
  Product2/1 -> W->Kw1/1
  W->Kw1/1 -> Add2/2, "  整车需求制动功率"/1
  Demux/3 -> m/s->kmph1/1
  Demux/2 -> 可用制动力/1
  Mux1/1 -> "  车速"/1, 车速跟随/1
  Add2/1 -> "  整车需求功率"/1

== system nonPred_TestModel_FCEV_ECMS_and_Battery_age/模式切换 ==
  note: 实际未使用
  .5 : Constant  Value=FC_power_min_kW
  .6 : Constant  Value=Bat_SOC_min
  .7 : Constant  Value=FC_power_max_kW
  .8 : Constant  Value=Bat_SOC_max
  Chart : Stateflow chart  TreatAsAtomicUnit=on
  Display3 : Display
  Scope : Scope
  To Workspace1 : ToWorkspace  VariableName=Mode  SampleTime=-1
  tag scope: Mode=global
  wires:
  Chart/1(Mode) -> Display3/1, [Mode], To Workspace1/1, Scope/1
  .6/1 -> Chart/2(Bat_SOC_min)
  .7/1 -> Chart/5(FC_power_max_kW)
  .5/1 -> Chart/4(FC_power_min_kW)
  .8/1 -> Chart/3(Bat_SOC_max)
  [Bat_SOC] -> Chart/6(Bat_SOC)
  [PS_power_dri_kW] -> Chart/1(PS_power_req_kW)

== system nonPred_TestModel_FCEV_ECMS_and_Battery_age/电池模型 ==
  note: Electrical Model
  note: Thermal Model (Cell)
  power req'd into bus (kW) : Inport
  Capacity Degradation Model (Cell) : Subsystem
  Electrical Model : Subsystem  Tag=electrical
  Gain : Gain  Gain=0.5
  Thermal Model : Subsystem
  Ts+Tc(℃) : Sum
  kW->W : Gain  Gain=1000  SaturateOnIntegerOverflow=on  OutDataTypeStr=Inherit: Same as input  ParamDataTypeStr=Inherit: Same as input
  温度(℃) : Scope
  电池需求输出功率(kW) : Scope
  Pb,ava : Outport  InitialOutput=0
  BattSoc : Outport  Port=2  InitialOutput=0
  wires:
  Thermal Model/1(Tc.) -> Ts+Tc(℃)/1
  Ts+Tc(℃)/1 -> Gain/1
  Thermal Model/2(Ts.) -> Ts+Tc(℃)/2
  Electrical Model/4(Pb,ava) -> Pb,ava/1
  Electrical Model/2(SOC) -> BattSoc/1, Capacity Degradation Model (Cell)/2(SOC)
  Electrical Model/3(I) -> Capacity Degradation Model (Cell)/3(I(A))
  Gain/1 -> Electrical Model/1(T), 温度(℃)/1, Capacity Degradation Model (Cell)/1(Temp (oC))
  Electrical Model/1(Qb) -> Thermal Model/1(Qb)
  kW->W/1 -> Electrical Model/2(Pb,r)
  power req'd into bus (kW)/1 -> 电池需求输出功率(kW)/1, kW->W/1

== system nonPred_TestModel_FCEV_ECMS_and_Battery_age/能量管理策略 (CD//CS) ==
  in kW : Inport
  Data Type Conversion : DataTypeConversion  SaturateOnIntegerOverflow=off  RndMeth=Floor
  FC on : Subsystem
  "FC pwr command, w/ limits enforced" : Subsystem
  Power command modified by SOC : Subsystem
  Power req'd from FC+DC/DC (kW) : Subsystem
  Product : Product  Inputs=3
  Relational Operator : RelationalOperator
  FC on1 : Outport
  FC power kW : Outport  Port=2
  wires:
  Power req'd from FC+DC/DC (kW)/1(pwr req'd of FC (W)) -> Power command modified by SOC/2(DC/DC+FC_pwr kW 2)
  in kW/1 -> FC on/4(bus pwr req), Power command modified by SOC/3(DC/DC+FC_pwr (kW)), Relational Operator/1, Power req'd from FC+DC/DC (kW)/1(power req'd by bus (W))
  Power command modified by SOC/1(FC power output req'd to FC (kW)) -> FC on/3(FC pwr command), "FC pwr command, w/ limits enforced"/3(FC pwr command)
  Relational Operator/1 -> FC on/1(ess max pwr would be insufficient), "FC pwr command, w/ limits enforced"/1(ess max pwr would be insufficient)
  Product/1 -> FC power kW/1
  [Bat_SOC] -> FC on/2(SOC), "FC pwr command, w/ limits enforced"/2(SOC), Power command modified by SOC/1(SOC)
  "FC pwr command, w/ limits enforced"/1(limited FC pwr command (W)) -> Product/2
  FC on/1(FC on) -> Data Type Conversion/1, FC on1/1
  Data Type Conversion/1 -> Product/3
  [Bat_power_dis_max_kW] -> Relational Operator/2
  [Bat_charge_sustaining_on] -> Product/1

== system nonPred_TestModel_FCEV_ECMS_and_Battery_age/车轮模型 ==
  "tractive force, brake force and speed req'd of tire/road interface 需求驱动力N 目标车速m/s 需求制动力N" : Inport
  "drive torque (Nm) brake torque (Nm) speed (rad/s) available from drivetrain into axle " : Inport  Port=2
  - : Gain  Gain=Veh_wheel_radius_m
  Add : Sum
  Add1 : Sum
  Add2 : Sum  Inputs=-+
  Add3 : Sum  Inputs=-+
  Constant : Constant  Value=0
  Demux : Demux  Outputs=3
  Demux1 : Demux  Outputs=3
  Gain1 : Gain  Gain=Veh_wheel_radius_m
  Gain2 : Gain  Gain=1/Veh_wheel_radius_m
  Gain3 : Gain  Gain=1/Veh_wheel_radius_m
  Gain4 : Gain  Gain=Veh_wheel_radius_m
  Interia torque : Subsystem
  Interia torque1 : Subsystem
  Mux : Mux  Inputs=3
  Mux3 : Mux  Inputs=3
  Regenerative energy compute : Subsystem
  Saturation : Saturate  UpperLimit=inf  LowerLimit=0
  Saturation1 : Saturate  UpperLimit=0  LowerLimit=-inf
  Scope : Scope
  Switch1 : Switch  Criteria=u2 > Threshold  Threshold=15  SaturateOnIntegerOverflow=off  InputSameDT=off
  Tire slip model : Subsystem
  Tire slip model1 : Subsystem
  axle input speed (rad/s) : Gain  Gain=1/Veh_wheel_radius_m
  drive torque (Nm) speed (rad/s) brake torque (Nm) req'd from drivetrain into axle : Outport  InitialOutput=0
  tractive force (N) brake force (N) linear speed achievable (m/s) : Outport  Port=2  InitialOutput=0
  wires:
  Demux/1 -> Gain1/1
  "tractive force, brake force and speed req'd of tire/road interface 需求驱动力N 目标车速m/s 需求制动力N"/1 -> Demux/1
  "drive torque (Nm) brake torque (Nm) speed (rad/s) available from drivetrain into axle "/1 -> Demux1/1
  Demux1/1 -> Add2/2
  Mux/1 -> drive torque (Nm) speed (rad/s) brake torque (Nm) req'd from drivetrain into axle/1
  Gain1/1 -> Add/2
  Add/1 -> Mux/1
  Add2/1 -> Gain2/1
  Gain2/1 -> Tire slip model/1(In1)
  Mux3/1 -> Scope/1, tractive force (N) brake force (N) linear speed achievable (m/s)/1
  Demux/2 -> axle input speed (rad/s)/1, Interia torque/1(车轮线速度 m/s), Interia torque1/1(车轮线速度 m/s)
  Interia torque/1(inertia torque (Nm)) -> Add2/1, Add/1
  Demux/3 -> Gain4/1
  Gain4/1 -> Add1/1
  Interia torque1/1(inertia torque (Nm)) -> Add3/1, Add1/2
  axle input speed (rad/s)/1 -> Switch1/2, Mux/2
  Switch1/1 -> Mux/3
  Constant/1 -> Switch1/3
  Add1/1 -> Switch1/1
  Saturation/1 -> Mux3/1
  Tire slip model/1(dri_force available in front wheel n) -> Saturation/1
  Tire slip model1/1(brk_force available in front wheel n) -> Saturation1/1
  Saturation1/1 -> Regenerative energy compute/1(motor brk force), Mux3/2
  Gain3/1 -> Tire slip model1/1(In1)
  Demux1/2 -> Add3/2
  Add3/1 -> Gain3/1
  Demux1/3 -> -/1
  -/1 -> Regenerative energy compute/3(spd2), Regenerative energy compute/2(spd), Mux3/3

== system nonPred_TestModel_FCEV_ECMS_and_Battery_age/车速 ==
  "  " : ToWorkspace  VariableName=Trip_distance_travelled_km  SampleTime=-1
  "  加速度" : ToWorkspace  VariableName=a_actual_k  SampleTime=-1
  "  车速" : ToWorkspace  VariableName=v_actual_k  SampleTime=-1
  Derivative : Derivative
  Display : Display
  Drive Cycle Source : autolibshared/Drive Cycle Source  cycleVar=Workspace variable  wsVar=DrvCycVps  fileVar=cycleFTP75.mat  tfinal="7031  seconds"  cycleRepeat=off  outAccPort=off  outGearPort=off  gearList=No gear data  t_wot1=5  xdot_woto=0  xdot_wot1=30  t_wot2=20  xdot_wot2=0  t_wotend=30  srcUnit=m/s  outUnit=m/s  srcAccUnit=m/s/s  outAccUnit=m/s^2  dt=1  aMode=1  faultOption=off  velBnd=2  velBndUnit=mph  inUnit=m/s  timeBnd=1  failOption=off  stopSim=off  maxFaultCnt=10  maxFaultTime=2  maxTotFaultTime=15  traceOption=off  dtTrace=1  traceWindow=10  lastDCname=Custom Data Set  lastOutUnit=mph  lastDT=1  lastTB=1  lastSB=2  forceCalcBound=off
  Integrator : Integrator
  Scope : Scope
  km/h->m/s : Gain  Gain=1/3.6
  km/h->m/s1 : Gain  Gain=3.6
  kmph-kmps : Gain  Gain=1/3600
  v_req(k) : Outport
  tag scope: Trip_distance_travelled_km=global
  wires:
  Drive Cycle Source/1 -> km/h->m/s1/1
  km/h->m/s/1 -> Derivative/1
  kmph-kmps/1 -> Integrator/1
  Derivative/1 -> "  加速度"/1
  Integrator/1 -> [Trip_distance_travelled_km], Display/1, "  "/1
  km/h->m/s1/1 -> kmph-kmps/1, km/h->m/s/1, Scope/1, "  车速"/1, v_req(k)/1

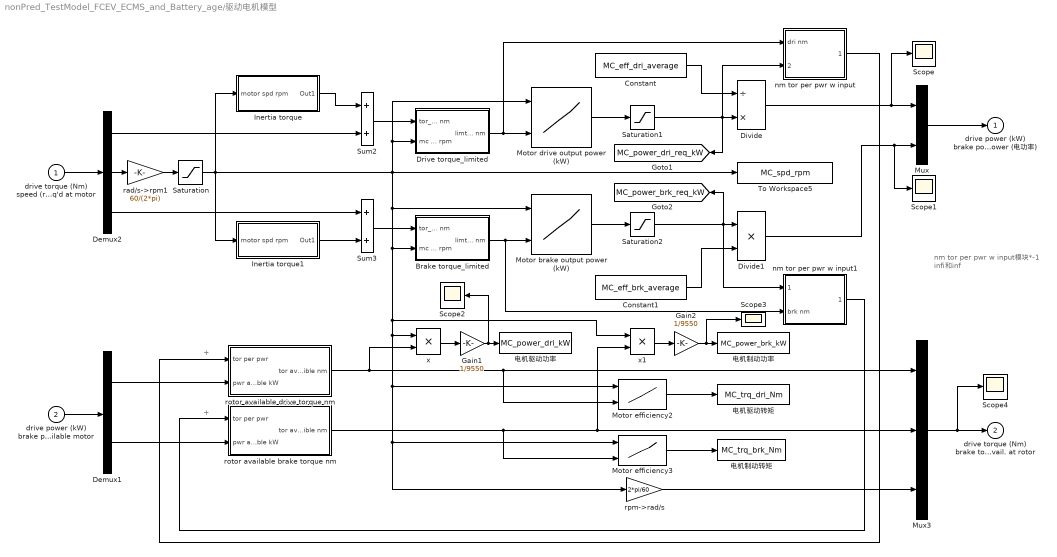
== system nonPred_TestModel_FCEV_ECMS_and_Battery_age/驱动电机模型 ==
  note: +
  note: +
  note: nm tor per pwr w input模块*-1
      | infi和inf
  drive torque (Nm) speed (rad/s) brake torque (Nm) req'd at motor : Inport
  drive power (kW) brake power (kW) input available motor : Inport  Port=2
  Brake torque_limited : Subsystem
  Constant : Constant  Value=MC_eff_dri_average
  Constant1 : Constant  Value=MC_eff_brk_average
  Demux1 : Demux  Outputs=2
  Demux2 : Demux  Outputs=3
  Divide : Product  Inputs=/*
  Divide1 : Product  Inputs=**
  Drive torque_limited : Subsystem
  Gain1 : Gain  Gain=1/9550
  Gain2 : Gain  Gain=1/9550
  Inertia torque : Subsystem
  Inertia torque1 : Subsystem
  Motor brake output power (kW) : Lookup2D  RowIndex=MC_ori_spd_rpm*MC_spd_scale  ColumnIndex=MC_ori_trq_brk_Nm*MC_trq_scale  Table=MC_ori_power_brk_req_kW*MC_spd_scale*MC_trq_scale
  Motor drive output power (kW) : Lookup2D  RowIndex=MC_ori_spd_rpm*MC_spd_scale  ColumnIndex=MC_ori_trq_dri_Nm*MC_trq_scale  Table=MC_ori_power_dri_req_kW*MC_spd_scale*MC_trq_scale
  Motor efficiency2 : Lookup2D  RowIndex=MC_ori_spd_rpm*MC_spd_scale  ColumnIndex=MC_ori_trq_Nm*MC_trq_scale  Table=MC_ori_eff*MC_spd_scale*MC_trq_scale
  Motor efficiency3 : Lookup2D  RowIndex=MC_ori_spd_rpm*MC_spd_scale  ColumnIndex=MC_ori_trq_Nm*MC_trq_scale  Table=MC_ori_eff*MC_spd_scale*MC_trq_scale
  Mux : Mux  Inputs=2
  Mux3 : Mux  Inputs=3
  Saturation : Saturate  UpperLimit=MC_spd_max_rpm  LowerLimit=MC_spd_min_rpm
  Saturation1 : Saturate  UpperLimit=MC_power_max_kW  LowerLimit=0  LinearizeAsGain=off
  Saturation2 : Saturate  UpperLimit=0  LowerLimit=-MC_power_max_kW
  Scope{,1..4} (5 alike) : Scope
  Sum2 : Sum  InputSameDT=on  SaturateOnIntegerOverflow=on  OutDataTypeStr=Inherit: Same as first input
  Sum3 : Sum  InputSameDT=on  SaturateOnIntegerOverflow=on  OutDataTypeStr=Inherit: Same as first input
  To Workspace5 : ToWorkspace  VariableName=MC_spd_rpm  SampleTime=-1
  nm tor per pwr w input : Subsystem
  nm tor per pwr w input1 : Subsystem
  rad/s->rpm1 : Gain  Gain=60/(2*pi)
  rotor available brake torque nm : Subsystem
  rotor available drive torque nm : Subsystem
  rpm->rad/s : Gain  Gain=2*pi/60
  x : Product  Inputs=**
  x1 : Product  Inputs=**
  电机制动功率 : ToWorkspace  VariableName=MC_power_brk_kW  SampleTime=-1
  电机制动转矩 : ToWorkspace  VariableName=MC_trq_brk_Nm  SampleTime=-1
  电机驱动功率 : ToWorkspace  VariableName=MC_power_dri_kW  SampleTime=-1
  电机驱动转矩 : ToWorkspace  VariableName=MC_trq_dri_Nm  SampleTime=-1
  drive power (kW) brake power (kW) req'd motor input power (电功率) : Outport  InitialOutput=0
  drive torque (Nm) brake torque (Nm) speed avail (rad/s) avail. at rotor : Outport  Port=2  InitialOutput=0
  tag scope: MC_power_brk_req_kW=global, MC_power_dri_req_kW=global
  wires:
  drive torque (Nm) speed (rad/s) brake torque (Nm) req'd at motor/1 -> Demux2/1
  rad/s->rpm1/1 -> Saturation/1
  Demux2/2 -> rad/s->rpm1/1
  Demux2/1 -> Sum2/2
  Inertia torque/1(Out1) -> Sum2/1
  Sum2/1 -> Drive torque_limited/1(tor_req nm)
  Drive torque_limited/1(limted mc torque nm) -> Motor drive output power (kW)/2, nm tor per pwr w input/1(dri nm)
  Motor drive output power (kW)/1 -> Saturation1/1
  Constant/1 -> Divide/1
  Divide/1 -> Scope/1, Mux/1
  Mux/1 -> drive power (kW) brake power (kW) req'd motor input power (电功率)/1
  Demux2/3 -> Sum3/1
  Inertia torque1/1(Out1) -> Sum3/2
  Sum3/1 -> Brake torque_limited/1(tor_req nm)
  Motor brake output power (kW)/1 -> Saturation2/1
  Saturation2/1 -> [MC_power_brk_req_kW], nm tor per pwr w input1/1(pwr brk kW), Divide1/1
  Constant1/1 -> Divide1/2
  Divide1/1 -> Scope1/1, Mux/2
  drive power (kW) brake power (kW) input available motor/1 -> Demux1/1
  Saturation1/1 -> nm tor per pwr w input/2(pwr dri kW), [MC_power_dri_req_kW], Divide/2
  Demux1/1 -> rotor available drive torque nm/2(pwr available kW)
  nm tor per pwr w input/1(tor per pwr) -> rotor available drive torque nm/1(tor per pwr)
  Demux1/2 -> rotor available brake torque nm/2(pwr available kW)
  nm tor per pwr w input1/1(tor per pwr) -> rotor available brake torque nm/1(tor per pwr)
  rotor available brake torque nm/1(tor avaible nm) -> Motor efficiency3/2, x1/2, Mux3/2
  rotor available drive torque nm/1(tor avaible nm) -> Motor efficiency2/2, Mux3/1, x/2
  rpm->rad/s/1 -> Mux3/3
  Motor efficiency3/1 -> 电机制动转矩/1
  Motor efficiency2/1 -> 电机驱动转矩/1
  Brake torque_limited/1(limted mc torque nm) -> nm tor per pwr w input1/2(brk nm), Motor brake output power (kW)/2
  Gain1/1 -> Scope2/1, 电机驱动功率/1
  x/1 -> Gain1/1
  Gain2/1 -> Scope3/1, 电机制动功率/1
  x1/1 -> Gain2/1
  Saturation/1 -> Inertia torque1/1(motor spd rpm), x1/1, x/1, Motor efficiency2/1, Motor efficiency3/1, rpm->rad/s/1, Brake torque_limited/2(mc spd rpm), Motor brake output power (kW)/1, To Workspace5/1, Motor drive output power (kW)/1, Drive torque_limited/2(mc spd rpm), Inertia torque/1(motor spd rpm)
  Mux3/1 -> Scope4/1, drive torque (Nm) brake torque (Nm) speed avail (rad/s) avail. at rotor/1

== system nonPred_TestModel_FCEV_ECMS_and_Battery_age/Power bus/pwr judgement ==
  In1 : Inport
  Add2 : Sum
  Constant{5..6,9..10} (4 alike) : Constant  Value=0
  Relational Operator2 : RelationalOperator  Operator=>  OutDataTypeStr=boolean  InputSameDT=off
  Relational Operator3 : RelationalOperator  Operator=>  OutDataTypeStr=boolean  InputSameDT=off
  SOC_min : Constant  Value=Bat_SOC_cs_min
  Switch3 : Switch  Threshold=0.1  SaturateOnIntegerOverflow=off  InputSameDT=off
  Switch4 : Switch  Threshold=0.1  SaturateOnIntegerOverflow=off  InputSameDT=off
  Switch5 : Switch  SaturateOnIntegerOverflow=off  InputSameDT=off
  Out1 : Outport
  wires:
  Switch5/1 -> Add2/2
  Constant10/1 -> Switch5/3
  Switch4/1 -> Switch5/1
  Constant9/1 -> Switch4/3
  Relational Operator3/1 -> Switch4/2
  SOC_min/1 -> Relational Operator3/2
  Switch3/1 -> Add2/1
  Constant6/1 -> Switch3/1
  Relational Operator2/1 -> Switch3/2
  Constant5/1 -> Relational Operator2/2
  In1/1 -> Switch4/1, Switch5/2, Switch3/3, Relational Operator2/1
  Add2/1 -> Out1/1
  [Bat_SOC] -> Relational Operator3/1

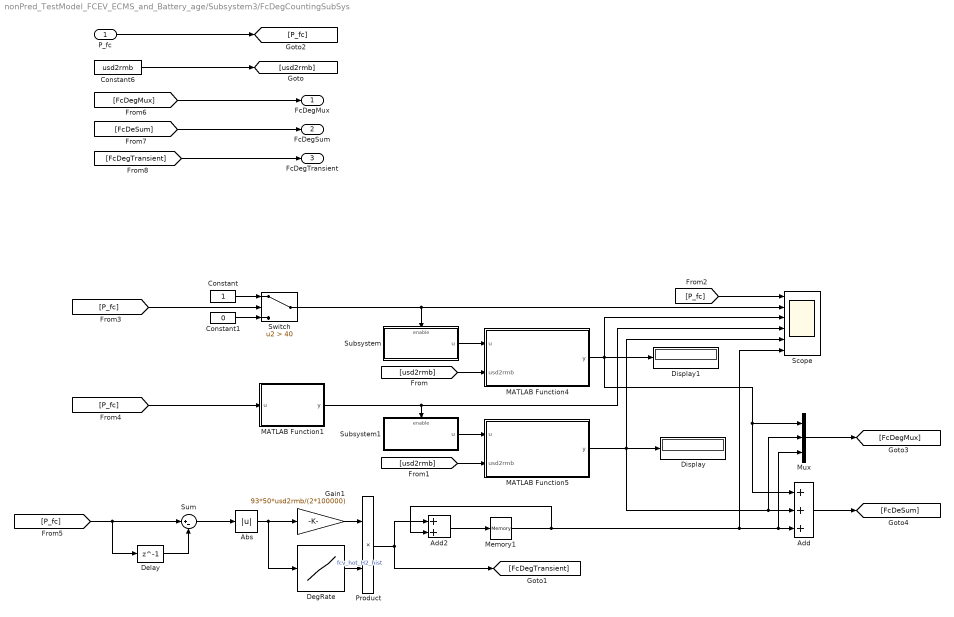
== system nonPred_TestModel_FCEV_ECMS_and_Battery_age/Subsystem3/FcDegCountingSubSys ==
  P_fc : Inport
  Abs : Abs  SaturateOnIntegerOverflow=off
  Add : Sum  Inputs=+++
  Add2 : Sum
  Constant : Constant
  Constant1 : Constant  Value=0
  Constant6 : Constant  Value=usd2rmb
  DegRate : Lookup_n-D  NumberOfTableDimensions=1  BreakpointsForDimension1=1:50  Table=tDegTable  RndMeth=Simplest
  Delay : Delay  DelayLength=1
  Display : Display
  Display1 : Display
  Gain1 : Gain  Gain=93*50*usd2rmb/(2*100000)
  MATLAB Function1 : MATLAB Function  TreatAsAtomicUnit=on
  MATLAB Function4 : MATLAB Function  TreatAsAtomicUnit=on
  MATLAB Function5 : MATLAB Function  TreatAsAtomicUnit=on
  Memory1 : Memory
  Mux : Mux  Inputs=3
  Product : Product
  Scope : Scope  NumInputPorts=6
  Subsystem : Subsystem
  Subsystem1 : Subsystem
  Sum : Sum  Inputs=|+-
  Switch : Switch  Criteria=u2 > Threshold  Threshold=40  SaturateOnIntegerOverflow=off  InputSameDT=off
  FcDegMux : Outport
  FcDegSum : Outport  Port=2
  FcDegTransient : Outport  Port=3
  wires:
  MATLAB Function5/1(y) -> Scope/5, Display/1, Mux/2, Add/2
  MATLAB Function1/1(y) -> Subsystem1/Enable, Scope/4
  Subsystem/1(u) -> MATLAB Function4/1(u)
  Constant/1 -> Switch/1
  [usd2rmb] -> MATLAB Function4/2(usd2rmb)
  Constant1/1 -> Switch/3
  [usd2rmb] -> MATLAB Function5/2(usd2rmb)
  Switch/1 -> Scope/2, Subsystem/Enable
  P_fc/1 -> [P_fc]
  Subsystem1/1(u) -> MATLAB Function5/1(u)
  MATLAB Function4/1(y) -> Scope/3, Mux/1, Add/1, Display1/1
  Constant6/1 -> [usd2rmb]
  [P_fc] -> Scope/1
  Memory1/1 -> Scope/6, Mux/3, Add/3, Add2/2
  Add2/1 -> Memory1/1
  Sum/1 -> Abs/1
  Abs/1 -> DegRate/1, Gain1/1
  Delay/1 -> Sum/2
  [P_fc] -> Delay/1, Sum/1
  [P_fc] -> Switch/2
  Add/1 -> [FcDeSum]
  Mux/1 -> [FcDegMux]
  [P_fc] -> MATLAB Function1/1(u)
  [FcDegMux] -> FcDegMux/1
  [FcDeSum] -> FcDegSum/1
  [FcDegTransient] -> FcDegTransient/1
  Product/1 -> [FcDegTransient], Add2/1
  Gain1/1 -> Product/1
  DegRate/1 -> Product/2  "fcv_hot_H2_hist"

== system nonPred_TestModel_FCEV_ECMS_and_Battery_age/Subsystem3/Fuel Rate Calculation1 ==
  note: Transient load response
  fc pwr : Inport
  "FC hydrogen consumption rate " : Lookup_n-D  NumberOfTableDimensions=1  BreakpointsForDimension1=FC_ori_power_kW  Table=FC_ori_fuel_rate_gps  RndMeth=Simplest
  fcv_H2_rate (g/s)1 : Outport
  wires:
  fc pwr/1 -> "FC hydrogen consumption rate "/1
  "FC hydrogen consumption rate "/1 -> fcv_H2_rate (g/s)1/1  "fcv_hot_H2_hist"

== system nonPred_TestModel_FCEV_ECMS_and_Battery_age/Subsystem3/Fuel cell efficiency calculation ==
  note: Carryover
  note: Transient load response
  fc power : Inport
  "FC efficiency " : Lookup_n-D  NumberOfTableDimensions=1  BreakpointsForDimension1=FC_ori_power_kW  Table=FC_ori_eff  RndMeth=Simplest
  "fc_eff " : Outport
  wires:
  "FC efficiency "/1 -> "fc_eff "/1
  fc power/1 -> "FC efficiency "/1

== system nonPred_TestModel_FCEV_ECMS_and_Battery_age/Subsystem3/Power Calculation ==
  note: Transient load response
  fc on : Inport
  Power command (kW) : Inport  Port=2
  "   " : Constant  Value=0
  Switch2 : Switch  Threshold=0.5
  Power output (kW) : Outport
  wires:
  "   "/1 -> Switch2/3
  Power command (kW)/1 -> Switch2/1
  fc on/1 -> Switch2/2
  Switch2/1 -> Power output (kW)/1

== system nonPred_TestModel_FCEV_ECMS_and_Battery_age/主减及变速器模型/ Effect of inertia (Nm)1 ==
  In1 : Inport
  Constant : Constant  Value=0
  Derivative : Derivative
  Switch : Switch  SaturateOnIntegerOverflow=off  InputSameDT=off
  inertia : Gain  Gain=Veh_final_drive_inertia
  Out1 : Outport
  wires:
  inertia/1 -> Out1/1
  In1/1 -> Derivative/1
  Derivative/1 -> Switch/3, Switch/2
  Constant/1 -> Switch/1
  Switch/1 -> inertia/1

== system nonPred_TestModel_FCEV_ECMS_and_Battery_age/主减及变速器模型/Effect of inertia (Nm) ==
  note: The inertia torque is the input torque required to accelerate the
      | final drive's inertia as measured on the input side.
  fd input speed (rad/s) : Inport
  Gain : Gain  Gain=Veh_final_drive_inertia  SaturateOnIntegerOverflow=on  OutDataTypeStr=Inherit: Same as input  ParamDataTypeStr=Inherit: Same as input
  d/dt : Derivative
  drag torque (Nm) : Outport  InitialOutput=0
  wires:
  fd input speed (rad/s)/1 -> d/dt/1
  d/dt/1 -> Gain/1
  Gain/1 -> drag torque (Nm)/1

== system nonPred_TestModel_FCEV_ECMS_and_Battery_age/主减及变速器模型/loss (Nm) ==
  note: The loss torque is zero when the gears are not turning,
      | and is applied at the input side of the gear reduction.
  "drive torque (Nm) " : Inport
  Add : Sum  Inputs=+-
  Gain : Gain  Gain=1/Veh_mech_eff
  Gain1 : Gain  Gain=1/Veh_final_drive_ratio
  drag torque (Nm) : Outport  InitialOutput=0
  wires:
  Add/1 -> drag torque (Nm)/1
  "drive torque (Nm) "/1 -> Gain1/1
  Gain1/1 -> Add/2, Gain/1
  Gain/1 -> Add/1

== system nonPred_TestModel_FCEV_ECMS_and_Battery_age/主减及变速器模型/loss (Nm)1 ==
  note: The loss torque is zero when the gears are not turning,
      | and is applied at the input side of the gear reduction.
  "drive torque (Nm) " : Inport
  Add : Sum  Inputs=+-
  Gain : Gain  Gain=1/Veh_mech_eff
  Gain1 : Gain  Gain=1/Veh_final_drive_ratio
  drag torque (Nm) : Outport  InitialOutput=0
  wires:
  Add/1 -> drag torque (Nm)/1
  "drive torque (Nm) "/1 -> Gain1/1
  Gain1/1 -> Add/2, Gain/1
  Gain/1 -> Add/1
